simulink model "statespacetest"  (R2018b)
settings: Solver=VariableStepAuto  StartTime=0.0  StopTime=1  RelTol=1e-3
values from neighbouring files (symbols this model uses):
  A_motor = [-R/L -Kv/L; Kt/J -b/J]    [motor_parameters.m]
  b = (Kt * average_current) / angular_velocity    [motor_parameters.m]
  B_motor = [1/L; 0]    [motor_parameters.m]
  C_motor = [1 0; 0 1]    [motor_parameters.m]
  D_motor = [0; 0]    [motor_parameters.m]
  J = rotor_inertia    (= 0.001785375)    [motor_parameters.m]
  Kt = current_data \ ((1e-3 * 9.81 * arm_length) .* mass_data)    [motor_parameters.m]
  Kv = 0.2915    [motor_parameters.m]
  L = R*rising_time    (= 0.00188546099291)    [motor_parameters.m]
  motor_supply_voltage = 12    [motor_parameters.m]
  R = eye(3) .* 1e-6    [KalmanFilter.m]    (also in motor_parameters.m = 1.45035460993)
  Ts_motor = 20e-6    (= 2e-05)    [motor_parameters.m]
undefined symbols (not defined in the file or in its folder): Down, Gain_motor, Up
libraries: powerlib x7, pePwmGenerator x1, cstblocks x1
settings Model: Creator=sasrinivas  LastModifiedBy=sasrinivas
settings SolverCC: ZeroCrossAlgorithm=Adaptive
settings DebuggingCC: IgnoredZcDiagnostic=none

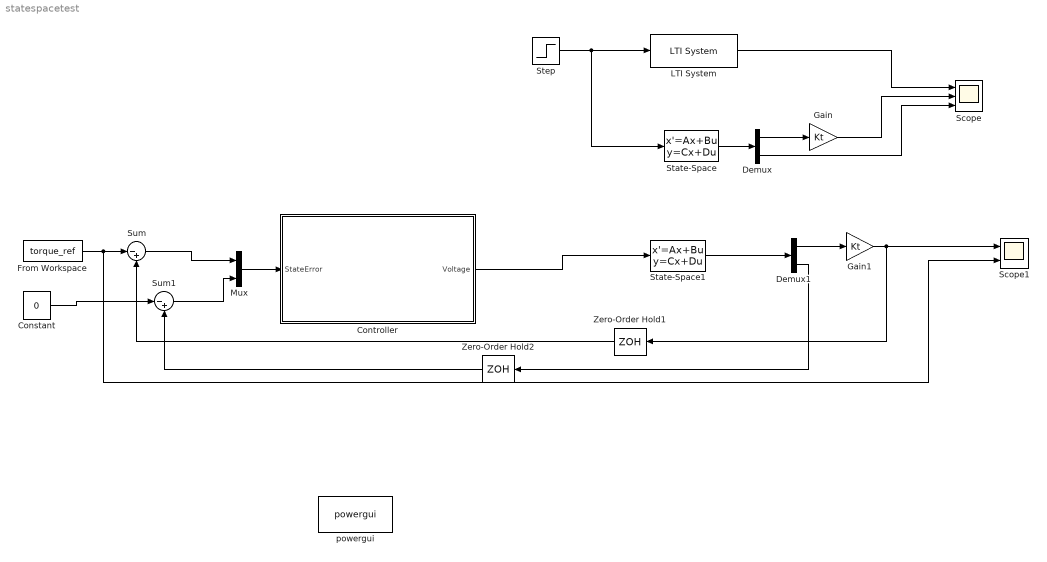
== system statespacetest ==
  Constant : Constant  Value=0
  Controller : Subsystem
  Demux : Demux  Outputs=2
  Demux1 : Demux  Outputs=2
  From Workspace : FromWorkspace  VariableName=torque_ref  SampleTime=0  Interpolate=off  OutputAfterFinalValue=Holding final value
  Gain : Gain  Gain=Kt
  Gain1 : Gain  Gain=Kt
  LTI System : cstblocks/LTI System  sys=torque_tf  IC=[]
  Mux : Mux  Inputs=2
  Scope : Scope  NumInputPorts=3
  Scope1 : Scope  NumInputPorts=2
  State-Space : StateSpace  A=[-R/L -Kv/L; Kt/J -b/J]  B=[1/L;0]  C=[1 0; 0 1]  D=[0; 0]  InitialCondition=0  ContinuousStateAttributes=['current', 'velocity']
  State-Space1 : StateSpace  A=A_motor  B=B_motor  C=C_motor  D=D_motor  InitialCondition=0  ContinuousStateAttributes=['current', 'velocity']
  Step : Step  Time=0.1  After=12  SampleTime=0
  Sum : Sum  Inputs=|-+
  Sum1 : Sum  Inputs=|-+
  Zero-Order Hold1 : ZeroOrderHold  SampleTime=Ts_motor
  Zero-Order Hold2 : ZeroOrderHold  SampleTime=Ts_motor
  powergui : powerlib/powergui  Priority=1  SimulationMode=Continuous  SampleTime=50e-6  frequency=60  Iterations=50  frequencyindice=0  Pbase=100e6  ErrMax=1e-4  UnitsV=kV  UnitsW=MW  buscounter=0  FunctionMessages=off  echomessages=off  EnableUseOfTLC=off  CurrentSourceSwitches=off  DisableSnubberDevices=off  DisableRonSwitches=off  DisableVfSwitches=off  DisplayEquations=off  SolverType=Tustin/Backward Euler (TBE)  Interpol=off  ExternalGateDelay=off  methode=off  Ts=100  x0status=blocks  SPID=on  SwTol=0  HookPort=off  RestoreLinks=warning  ResistiveCurrentMeasurement=off  Frange=[0:2:500]  Ylog=off  Xlog=on  ShowGrid=off  save=off  variable=ZData  structure=0  ZoomFFT=off  StartTime=0.0  cycles=1  DisplayStyle=1  fundamental=60  FreqAxis=off  MaxFrequency=1000  frequencyindicesteady=1  RmsSteady=1  display=off
  wires:
  Step/1 -> State-Space/1, LTI System/1
  LTI System/1 -> Scope/1
  State-Space/1 -> Demux/1
  Demux/1 -> Gain/1
  Gain/1 -> Scope/2
  Demux/2 -> Scope/3
  Gain1/1 -> Scope1/1, Zero-Order Hold1/1
  Demux1/1 -> Gain1/1
  State-Space1/1 -> Demux1/1
  From Workspace/1 -> Scope1/2, Sum/1
  Zero-Order Hold1/1 -> Sum/2
  Sum/1 -> Mux/1
  Mux/1 -> Controller/1(StateError)
  Constant/1 -> Sum1/1
  Sum1/1 -> Mux/2
  Demux1/2 -> Zero-Order Hold2/1
  Controller/1(Voltage) -> State-Space1/1
  Zero-Order Hold2/1 -> Sum1/2

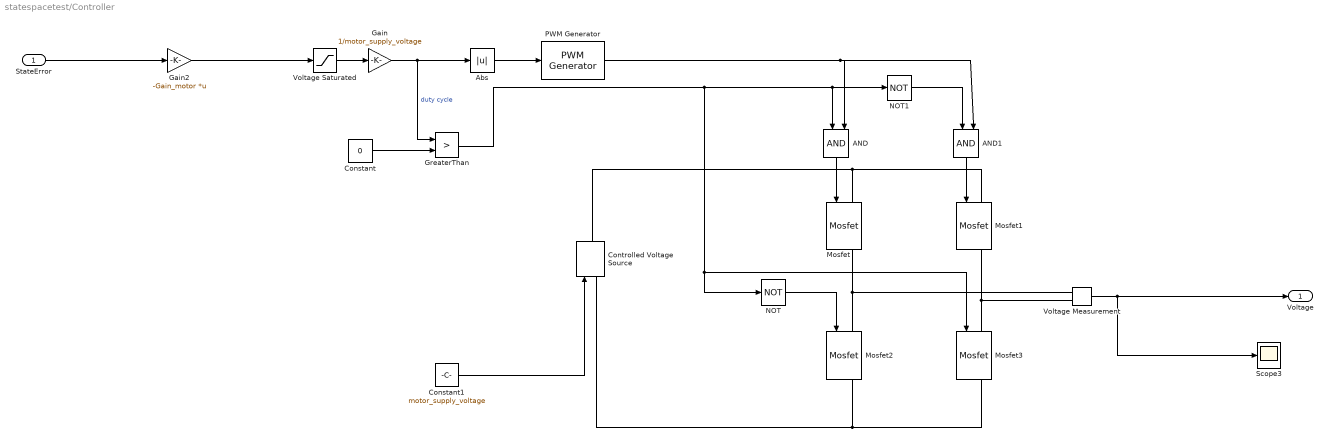
== system statespacetest/Controller ==
  StateError : Inport
  AND : Logic  IconShape=distinctive  AllPortsSameDT=off  OutDataTypeStr=boolean
  AND1 : Logic  IconShape=distinctive  AllPortsSameDT=off  OutDataTypeStr=boolean
  Abs : Abs
  Constant : Constant  Value=0
  Constant1 : Constant  Value=motor_supply_voltage
  Controlled Voltage Source : powerlib/Electrical Sources/Controlled Voltage Source  Initialize=on  Source_Type=DC  Amplitude=0  Phase=0  Frequency=0  Measurements=None
  Gain : Gain  Gain=1/motor_supply_voltage
  Gain2 : Gain  Gain=-Gain_motor  Multiplication=Matrix(K*u)
  GreaterThan : RelationalOperator  Operator=>  OutDataTypeStr=boolean  RndMeth=Simplest
  Mosfet{,1..3} (4 alike) : powerlib/Power Electronics/Mosfet  Ron=0.01  Lon=0  Rd=0.01  Vfd=0  IC=0  Rs=1e5  Cs=inf  Measurements=on
  NOT : Logic  Operator=NOT  IconShape=distinctive  AllPortsSameDT=off  OutDataTypeStr=boolean
  NOT1 : Logic  Operator=NOT  IconShape=distinctive  AllPortsSameDT=off  OutDataTypeStr=boolean
  PWM Generator : pePwmGenerator/PWM Generator  CarrCount=Up-Down  Tper=20e-6  Ts=1e-6
  Scope3 : Scope
  Voltage Measurement : powerlib/Measurements/Voltage Measurement  PhasorSimulation=off  OutputType=Complex  PSBequivalent=0
  Voltage Saturated : Saturate  UpperLimit=12  LowerLimit=-12
  Voltage : Outport
  wires:
  Constant1/1 -> Controlled Voltage Source/1
  PWM Generator/1 -> AND/2, AND1/2
  AND/1 -> Mosfet/1
  AND1/1 -> Mosfet1/1
  NOT1/1 -> AND1/1
  GreaterThan/1 -> Mosfet3/1, NOT/1, AND/1, NOT1/1
  Voltage Measurement/1 -> Scope3/1, Voltage/1
  Voltage Saturated/1 -> Gain/1
  NOT/1 -> Mosfet2/1
  Gain/1 -> GreaterThan/1, Abs/1  "duty cycle"
  Constant/1 -> GreaterThan/2
  Abs/1 -> PWM Generator/1
  StateError/1 -> Gain2/1
  Gain2/1 -> Voltage Saturated/1
  connections:
  Controlled Voltage Source/LConn1 -- Mosfet2/RConn1 -- Mosfet3/RConn1
  Controlled Voltage Source/RConn1 -- Mosfet1/LConn1 -- Mosfet/LConn1
  Mosfet/RConn1 -- Mosfet2/LConn1 -- Voltage Measurement/LConn1
  Mosfet1/RConn1 -- Voltage Measurement/LConn2 -- Mosfet3/LConn1
